simulink model "PSS2A"  (R2020a)
settings: Solver=ode8  StartTime=0.0  StopTime=5  FixedStep=0.005  MaxStep=0.005  RelTol=1e-3
undefined symbols (not defined in the file): K_S1, K_S2, K_S3, M, T_6, T_7, T_8, T_9, T_w1, T_w2, T_w3, T_w4, V_S1MAX, V_S1MIN, V_S2MAX, V_S2MIN, V_STMAX, V_STMIN
libraries: eeGeneralControl x10
settings Model: Creator=meagh  LastModifiedBy=meagh

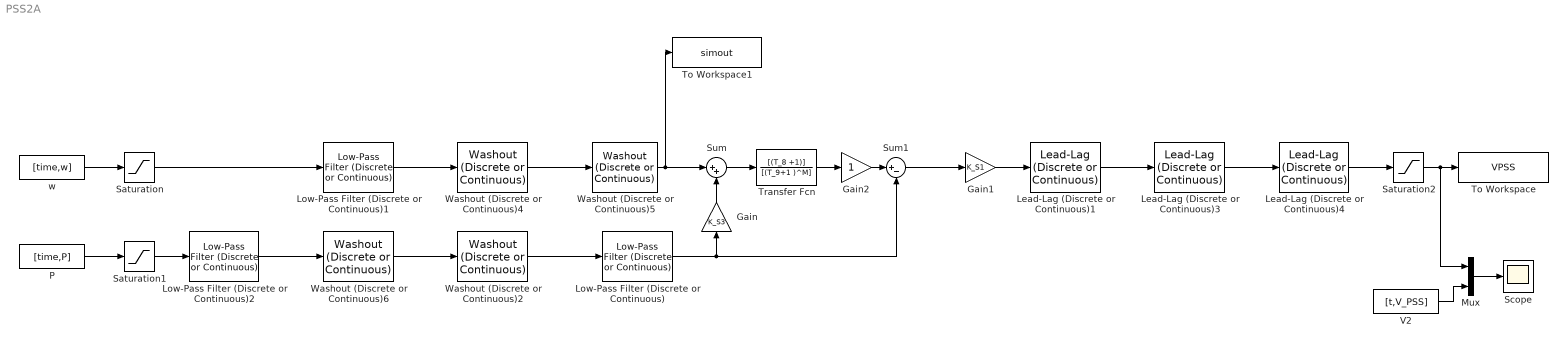
== system PSS2A ==
  Gain : Gain  Gain=K_S3
  Gain1 : Gain  Gain=K_S1
  Gain2 : Gain
  Lead-Lag (Discrete or Continuous)1 : eeGeneralControl/Lead-Lag (Discrete or Continuous)  T1=T_1  T2=T_2  B=inf  A=-inf  init_option=Inherited from block input  x0=0  Ts=0
      settings: SourceProductBaseCode=PS
  Lead-Lag (Discrete or Continuous)3 : eeGeneralControl/Lead-Lag (Discrete or Continuous)  T1=T_3  T2=T_4  B=inf  A=-inf  init_option=Inherited from block input  x0=0  Ts=0
      settings: SourceProductBaseCode=PS
  Lead-Lag (Discrete or Continuous)4 : eeGeneralControl/Lead-Lag (Discrete or Continuous)  T1=T_10  T2=T_11  B=inf  A=-inf  init_option=Inherited from block input  x0=0  Ts=0
      settings: SourceProductBaseCode=PS
  Low-Pass Filter (Discrete or Continuous) : eeGeneralControl/Low-Pass Filter (Discrete or Continuous)  K=K_S2  T=T_7  B=inf  A=-inf  init_option=Inherited from block input  x0=0  Ts=0
  Low-Pass Filter (Discrete or Continuous)1 : eeGeneralControl/Low-Pass Filter (Discrete or Continuous)  K=1  T=T_6  B=inf  A=-inf  init_option=Inherited from block input  x0=0  Ts=0
  Low-Pass Filter (Discrete or Continuous)2 : eeGeneralControl/Low-Pass Filter (Discrete or Continuous)  K=1  T=T_6  B=inf  A=-inf  init_option=Inherited from block input  x0=0  Ts=0
  Mux : Mux  Inputs=2
  P : FromWorkspace  VariableName=[time,P]
  Saturation : Saturate  UpperLimit=V_S1MAX  LowerLimit=V_S1MIN
  Saturation1 : Saturate  UpperLimit=V_S2MAX  LowerLimit=V_S2MIN
  Saturation2 : Saturate  UpperLimit=V_STMAX  LowerLimit=V_STMIN
  Scope : Scope
  Sum : Sum  Inputs=|++
  Sum1 : Sum  Inputs=|+-
  To Workspace : ToWorkspace  VariableName=VPSS  SaveFormat=Timeseries  SampleTime=-1
  To Workspace1 : ToWorkspace  VariableName=simout  SaveFormat=Timeseries  SampleTime=-1
  Transfer Fcn : TransferFcn  Numerator=[(T_8 +1)]  Denominator=[(T_9+1 )^M]
  V2 : FromWorkspace  VariableName=[t,V_PSS]
  Washout (Discrete or Continuous)2 : eeGeneralControl/Washout (Discrete or Continuous)  T=T_w4  init_option=Inherited from block input  x0=0  Ts=0
      settings: SourceProductBaseCode=PS
  Washout (Discrete or Continuous)4 : eeGeneralControl/Washout (Discrete or Continuous)  T=T_w1  init_option=Specify as parameter  x0=0  Ts=0
      settings: SourceProductBaseCode=PS
  Washout (Discrete or Continuous)5 : eeGeneralControl/Washout (Discrete or Continuous)  T=T_w2  init_option=Inherited from block input  x0=0  Ts=0
      settings: SourceProductBaseCode=PS
  Washout (Discrete or Continuous)6 : eeGeneralControl/Washout (Discrete or Continuous)  T=T_w3  init_option=Specify as parameter  x0=0  Ts=0
      settings: SourceProductBaseCode=PS
  w : FromWorkspace  VariableName=[time,w]
  wires:
  Gain/1 -> Sum/2
  Low-Pass Filter (Discrete or Continuous)/1 -> Sum1/2, Gain/1
  Sum/1 -> Transfer Fcn/1
  Sum1/1 -> Gain1/1
  Gain1/1 -> Lead-Lag (Discrete or Continuous)1/1
  Lead-Lag (Discrete or Continuous)1/1 -> Lead-Lag (Discrete or Continuous)3/1
  Lead-Lag (Discrete or Continuous)3/1 -> Lead-Lag (Discrete or Continuous)4/1
  Lead-Lag (Discrete or Continuous)4/1 -> Saturation2/1
  Saturation/1 -> Low-Pass Filter (Discrete or Continuous)1/1
  Saturation1/1 -> Low-Pass Filter (Discrete or Continuous)2/1
  Washout (Discrete or Continuous)2/1 -> Low-Pass Filter (Discrete or Continuous)/1
  Washout (Discrete or Continuous)5/1 -> Sum/1, To Workspace1/1
  Washout (Discrete or Continuous)6/1 -> Washout (Discrete or Continuous)2/1
  Washout (Discrete or Continuous)4/1 -> Washout (Discrete or Continuous)5/1
  Mux/1 -> Scope/1
  Saturation2/1 -> Mux/1, To Workspace/1
  V2/1 -> Mux/2
  Transfer Fcn/1 -> Gain2/1
  Gain2/1 -> Sum1/1
  P/1 -> Saturation1/1
  w/1 -> Saturation/1
  Low-Pass Filter (Discrete or Continuous)1/1 -> Washout (Discrete or Continuous)4/1
  Low-Pass Filter (Discrete or Continuous)2/1 -> Washout (Discrete or Continuous)6/1
